simulink model "DEV2P"  (R2023a)
settings: Solver=FixedStepAuto  StartTime=0.0  StopTime=2000  RelTol=1e-3
model workspace (MAT data in the model file):
  SampleTime = 0.001
  T_npxls = 4
  T_pupil = 100
  T_whisk = 20
  maxFrames = 1800000
  tStop = 1800
  toneDuration = 1.5
undefined symbols (not defined in the file or in its folder): Ended, Single
libraries: speedgoatlib_IO191 x3
settings Model: Creator=electro  LastModifiedBy=ahab
settings SolverCC: ConcurrentTasks=on  PositivePriorityOrder=on  AutoInsertRateTranBlk=on
settings DataIOCC: SaveFormat=Array
settings OptimizationCC: BlockReduction=off  OptimizeBlockIOStorage=off  EnhancedBackFolding=on  PassReuseOutputArgsThreshold=0  OptimizeBlockOrder=speed  DifferentSizesBufferReuse=on
settings DebuggingCC: TasksWithSamePriorityMsg=none  ParameterTunabilityLossMsg=error  SFUnexpectedBacktrackingDiag=warning  SFNoUnconditionalDefaultTransitionDiag=warning
settings HardwareCC: ProdBitPerLong=64  ProdLongLongMode=on  ProdHWDeviceType=Intel->x86-64 (Linux 64)
settings SFSimCC: SimUserIncludeDirs="\"/usr/local/MATLAB/R2023a/toolbox/slrealtime/target/kernel/dist/include/verify\""  MATLABDynamicMemAlloc=off
settings RTWCC: Description=Simulink Real-Time  SystemTargetFile=slrealtime.tlc  TemplateMakefile=slrealtime_default_tmf  GenerateReport=on  RTWVerbose=off  CustomInclude=/usr/local/MATLAB/R2023a/toolbox/slrealtime/target/kernel/dist/include,  Toolchain=Simulink Real-Time Toolchain  BuildConfiguration=Faster Runs  CodeExecutionProfiling=on  TargetLang=C++
settings CodeAppCC: ForceParamTrailComments=on  OperatorAnnotations=on  EnableCustomComments=on

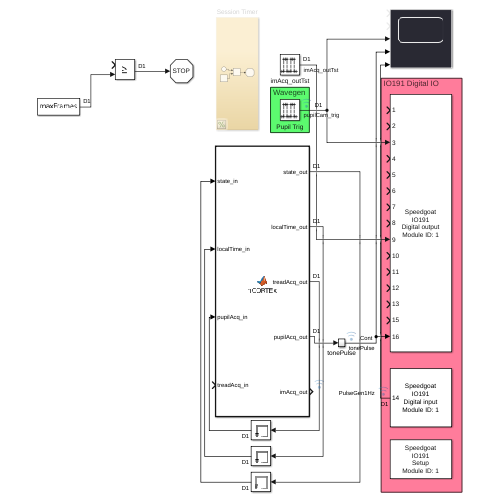
[thumbnail: Simulink's stored preview of the top-level diagram]
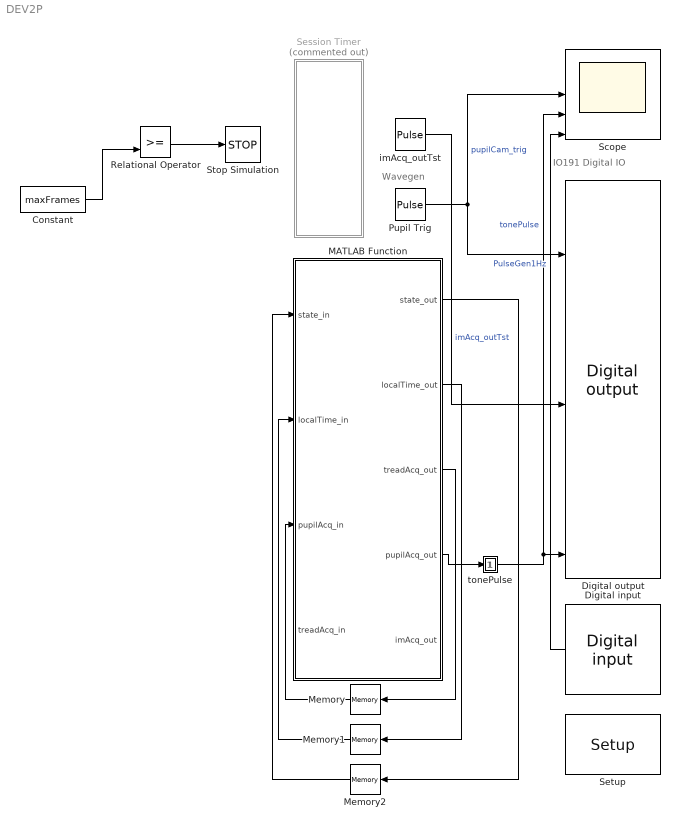
== system DEV2P ==
  note: IO191 Digital IO
  note: Wavegen
  Constant : Constant  Value=maxFrames  VectorParams1D=off  SampleTime=SampleTime
  "Digital input " : speedgoatlib_IO191/Digital input   parModuleId=1  parSampleTime=SampleTime  parPciSlot=-1  parDiChannels=14
      settings: SourceProductName=Simulink Real-Time: Speedgoat I/O Blockset
  "Digital output " : speedgoatlib_IO191/Digital output   parModuleId=1  parSampleTime=0.001  parPciSlot=-1  parDoChannels=[1 2 3 4 5 6 7 8 9 10 11 12 13 15 16]  parDoInitValues=[0 0 0 0 0 0 0 0 0 0 0 0 0 0 0]  parDoResets=[1 1 1 1 1 1 1 1 1 1 1 1 1 1 1]
      settings: SourceProductName=Simulink Real-Time: Speedgoat I/O Blockset
  MATLAB Function : MATLAB Function  TreatAsAtomicUnit=on
  Memory : Memory
  Memory1 : Memory
  Memory2 : Memory  InitialCondition=1
  Pupil Trig : DiscretePulseGenerator  Period=T_pupil  PulseWidth=T_pupil/2  SampleTime=SampleTime
  Relational Operator : RelationalOperator  OutDataTypeStr=boolean  RndMeth=Simplest  InputSameDT=off
  Scope : Scope  NumInputPorts=5
  Session Timer : Subsystem  Commented=on
  "Setup " : speedgoatlib_IO191/Setup   parModuleId=1  parPciSlot=-1  parTriggerSignal=TTL  parAdcChannels=[1 2]  parAdcRanges=[3 3]  parAdcChannel1=on  parAdcChannel2=on  parAdcChannel3=off  parAdcChannel4=off  parAdcChannel5=off  parAdcChannel6=off  parAdcChannel7=off  parAdcChannel8=off  parAdcMode=Single-Ended  parAdcRate=100000  parAdcRange11=+-10.24 V  parAdcRange21=+-24.576 V  parAdcRange12=+-10.24 V  parAdcRange22=+-24.576 V  parAdcRange13=+-10.24 V  parAdcRange23=+-24.576 V  parAdcRange14=+-10.24 V  parAdcRange24=+-24.576 V  parAdcRange15=+-10.24 V  parAdcRange25=+-24.576 V  parAdcRange16=+-10.24 V  parAdcRange26=+-24.576 V  parAdcRange17=+-10.24 V  parAdcRange27=+-24.576 V  parAdcRange18=+-10.24 V  parAdcRange28=+-24.576 V  parDacChannels=[1 2]  parDacChannel1=on  parDacChannel2=on  parDacChannel3=off  parDacChannel4=off  parDacMode=Single-Ended  parDacRanges=[4 4]  parDacInitValues=[0 0]  parDacResets=[1 1]  parDacRange1=+-10 V  parDacInitValue1=0  parDacReset1=on  parDacRange2=+-10 V  parDacInitValue2=0  parDacReset2=on  parDacRange3=+-10 V  parDacInitValue3=0  parDacReset3=on  parDacRange4=+-10 V  parDacInitValue4=0  parDacReset4=on  parDiChannels=14  parDoChannels=[1 2 3 4 5 6 7 8 9 10 11 12 13 15 16]  parDioFirstControl=[1 2 3 4 5 6 8 9]  parDioSecondControl=0  parDioChannel1=Out  parExtra1=I  parExtra2=I  parExtra3=I  parDioChannel2=Out  parDioChannel3=Out  parDioChannel4=Out  parDioChannel5=Out  parDioChannel6=Out  parDioChannel7=In  parDioChannel8=Out  parDioChannel9=Out  parDoInitValues=[0 0 0 0]  parDoResets=[1 1 1 1]  parDoInitValue1=0  parDoReset1=on  parDoInitValue2=0  parDoReset2=on  parDoInitValue3=0  parDoReset3=on  parDoInitValue4=0  parDoReset4=on  parDoInitValue5=0  parDoReset5=on  parDoInitValue6=0  parDoReset6=on  parDoInitValue7=0  parDoReset7=on  parDoInitValue8=0  parDoReset8=on  parDoInitValue9=0  parDoReset9=on  parDoInitValue10=0  parDoReset10=on  parDoInitValue11=0  parDoReset11=on  parDoInitValue12=0  parDoReset12=on  parDoInitValue13=0  parDoReset13=on  parDoInitValue14=0  parDoReset14=on  parDoInitValue15=0  parDoReset15=on  parDoInitValue16=0  parDoReset16=on
      settings: SourceProductName=Simulink Real-Time: Speedgoat I/O Blockset
  Stop Simulation : Stop
  imAcq_outTst : DiscretePulseGenerator  Period=5000  PulseWidth=2500  SampleTime=SampleTime
  tonePulse : Subsystem
  wires:
  Pupil Trig/1 -> Scope/3, "Digital output "/3  "pupilCam_trig"
  MATLAB Function/3(treadAcq_out) -> Memory/1
  Memory/1 -> MATLAB Function/3(pupilAcq_in)
  MATLAB Function/2(localTime_out) -> Memory1/1
  Memory1/1 -> MATLAB Function/2(localTime_in)
  MATLAB Function/1(state_out) -> Memory2/1
  Memory2/1 -> MATLAB Function/1(state_in)
  tonePulse/1(tonePulse) -> "Digital output "/15, Scope/4  "tonePulse"
  MATLAB Function/4(pupilAcq_out) -> tonePulse/1(onesetTone_trig)
  "Digital input "/1 -> Scope/5  "PulseGen1Hz"
  Relational Operator/1 -> Stop Simulation/1
  Constant/1 -> Relational Operator/2
  imAcq_outTst/1 -> "Digital output "/9  "imAcq_outTst"

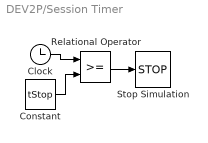
== system DEV2P/Session Timer ==
  Clock : Clock
      settings: Decimation=100
  Constant : Constant  Value=tStop  VectorParams1D=off  SampleTime=SampleTime
  Relational Operator : RelationalOperator  OutDataTypeStr=boolean  RndMeth=Simplest  InputSameDT=off
  Stop Simulation : Stop
  wires:
  Relational Operator/1 -> Stop Simulation/1
  Constant/1 -> Relational Operator/2
  Clock/1 -> Relational Operator/1

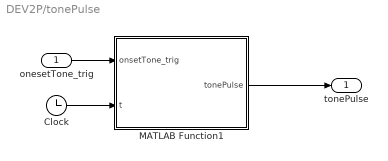
== system DEV2P/tonePulse ==
  onesetTone_trig : Inport
  Clock : Clock
  MATLAB Function1 : MATLAB Function  TreatAsAtomicUnit=on
  tonePulse : Outport
  wires:
  MATLAB Function1/1(tonePulse) -> tonePulse/1
  onesetTone_trig/1 -> MATLAB Function1/1(onsetTone_trig)
  Clock/1 -> MATLAB Function1/2(t)

== matlab function DEV2P/MATLAB Function ==
  data: state_in input; localTime_in input; pupilAcq_in input; treadAcq_in input; state_out output; localTime_out output; treadAcq_out output; pupilAcq_out output; imAcq_out output
function [state_out, localTime_out, treadAcq_out, pupilAcq_out, imAcq_out] = nCORTEx(state_in, localTime_in, pupilAcq_in, treadAcq_in)       
    
    % counter_out=counter_in+1;    
    switch (state_in)         
        % case {0} % LOAD SESSION PARAMS
            % params = loadSlParams;
            % state_out = 1;
        case {0}
            imAcq_out = 5;
            state_out = 2;
            localTime_out = localTime_in + 1;   
            pupilAcq_out = 1;
            treadAcq_out = 1;
        % case {1} %% TRIAL START grab 1800 frames
        %     imAcq_out = 5;
        %     pupilAcq_out = 1;
        %     treadAcq_out = 1;
        %     if framesAcq > 1800
        %         state_out = 2;
        %     end

        case {2} %% RESTING - dont collect anything
            % imAcq_out=imAcq_in;
            imAcq_out = 0;
            pupilAcq_out = pupilAcq_in;
            treadAcq_out = treadAcq_in;
            localTime_out = localTime_in + 1;
            % LEDStimTrig = 1
            % whiskerStimTrig = 1

            state_out = state_in;

            % if % done nothing for long enough
            %     state_out = 3;
            % end

        % case {3}
        %     % start whisker stim
        %     whiskerStimTrig = 1;
        %     % then start LED sto,
        %     % then do both
        % 
        otherwise            
            state_out = state_in;
            localTime_out = localTime_in;        
            pupilAcq_out = pupilAcq_in;
            treadAcq_out = treadAcq_in;
            imAcq_out = 0;
    end          
    
end

== matlab function DEV2P/tonePulse/MATLAB Function1 ==
  data: onsetTone_trig input; tonePulse output; t input
function tonePulse  = holdTone(onsetTone_trig, t) 
    % When the trigger onsetTone_trig is received, it sets tonePulse to 1 and 
    % stores the current time t in the persistent variable t0.   
    
    % If the trigger is not received (onsetTone_trig is false), it checks whether t0 is not 
    % empty (indicating that a trigger has been received previously). 
    % If t0 is not empty, it checks if (t - t0) is less than 1.5 seconds. 
    % If so, it keeps tonePulse set to 1, maintaining the tone pulse for 1.5 seconds after the trigger. 
    
    % After 1.5 seconds have passed since the trigger was received (when (t - t0) is 
    % greater than or equal to 1.5 seconds), it clears the persistent variable 
    % t0, effectively resetting it to its initial condition.     
    
    persistent t0;
    if onsetTone_trig                
        tonePulse = 1; % set tone pulse high until 1.5 s elapses            
        t0 = t; % store current time 
    elseif ~isempty(t0) 
        if (t - t0) < 1.5
            tonePulse = 1;
        else
            tonePulse = 0;
            clear t0 % reset t0 to initial condition
        end        
    else % reset to 0 if no more trigger activity
        tonePulse = 0;        
    end
end
